simulink model "modelo_diagrama_simulacion_observador"  (Simulink 8.5)
settings: Solver=ode45  StartTime=0.0  StopTime=10  RelTol=1e-3
undefined symbols (not defined in the file): G, Ts
settings Model: Creator=n221  LastModifiedBy=ARTURO  CovModelRefEnable=off
settings DataIOCC: SaveFormat=Dataset  SignalLoggingSaveFormat=Dataset
settings OptimizationCC: ExpressionDepthLimit=128
settings DebuggingCC: UnderspecifiedInitializationDetection=Simplified  MergeDetectMultiDrivingBlocksExec=error  FcnCallInpInsideContextMsg=EnableAllAsError  StateNameClashWarn=none
settings HardwareCC: ProdBitPerPointer=64  ProdLargestAtomicFloat=Float  ProdIntDivRoundTo=Zero  ProdEndianess=LittleEndian  ProdHWDeviceType=Specified
settings GRTTargetCC: GeneratePreprocessorConditionals=Use local settings  CombineOutputUpdateFcns=on  GRTInterface=off

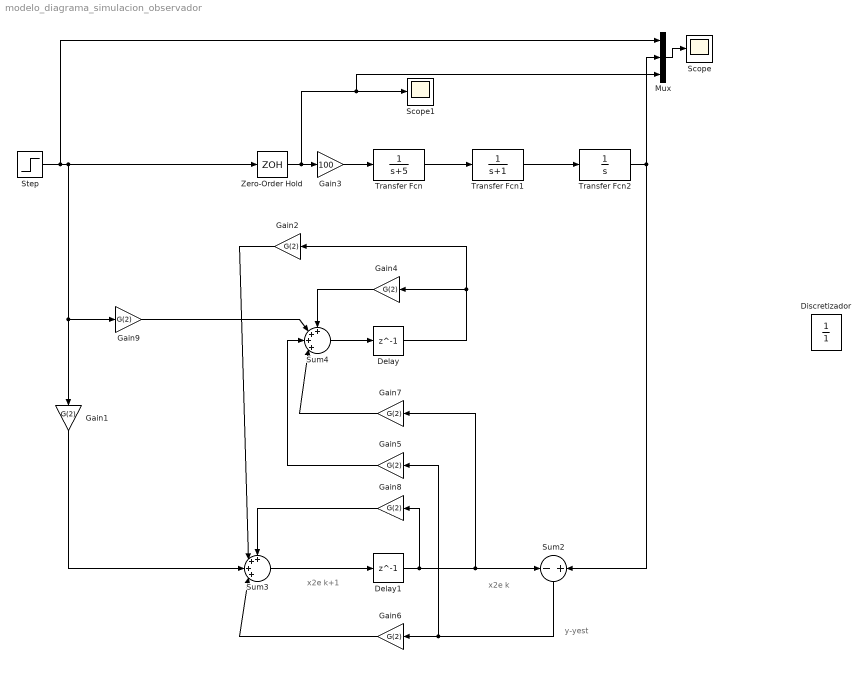
== system modelo_diagrama_simulacion_observador ==
  note: x2e k+1
  note: x2e k
  note: y-yest
  Delay : Delay  DelayLength=1  SampleTime=Ts
  Delay1 : Delay  DelayLength=1  SampleTime=Ts
  Discretizador : DiscreteTransferFcn  Denominator=[1]  SampleTime=Ts
  Gain{1..2,4..9} (8 alike) : Gain  Gain=G(2)
  Gain3 : Gain  Gain=100
  Mux : Mux  Inputs=3
  Scope : Scope
      settings: YMin=-0.19955  YMax=1.18155  SaveName=datos
  Scope1 : Scope
      settings: YMin=-0.13963  YMax=0.64227
  Step : Step  Time=0  SampleTime=Ts
  Sum2 : Sum  Inputs=-|+
  Sum3 : Sum  Inputs=++++|
  Sum4 : Sum  Inputs=++++|
  Transfer Fcn : TransferFcn  Denominator=[1 5]
  Transfer Fcn1 : TransferFcn  Denominator=[1 1]
  Transfer Fcn2 : TransferFcn  Denominator=[1 0]
  Zero-Order Hold : ZeroOrderHold  SampleTime=Ts
  wires:
  Transfer Fcn1/1 -> Transfer Fcn2/1
  Transfer Fcn/1 -> Transfer Fcn1/1
  Step/1 -> Mux/1, Gain1/1, Gain9/1, Zero-Order Hold/1
  Transfer Fcn2/1 -> Sum2/2, Mux/2
  Zero-Order Hold/1 -> Mux/3, Scope1/1, Gain3/1
  Gain3/1 -> Transfer Fcn/1
  Mux/1 -> Scope/1
  Sum2/1 -> Gain5/1, Gain6/1
  Delay1/1 -> Gain8/1, Gain7/1, Sum2/1
  Gain6/1 -> Sum3/4
  Sum3/1 -> Delay1/1
  Sum4/1 -> Delay/1
  Gain1/1 -> Sum3/3
  Gain7/1 -> Sum4/4
  Gain5/1 -> Sum4/3
  Gain2/1 -> Sum3/2
  Gain8/1 -> Sum3/1
  Gain4/1 -> Sum4/1
  Gain9/1 -> Sum4/2
  Delay/1 -> Gain2/1, Gain4/1
